simulink model "assignmentJoint"  (R2021b)
settings: Solver=VariableStepAuto  StartTime=0.0  StopTime=10.0  MaxStep=0.02  RelTol=1e-3
settings Model: Creator=emil1  LastModifiedBy=emil1

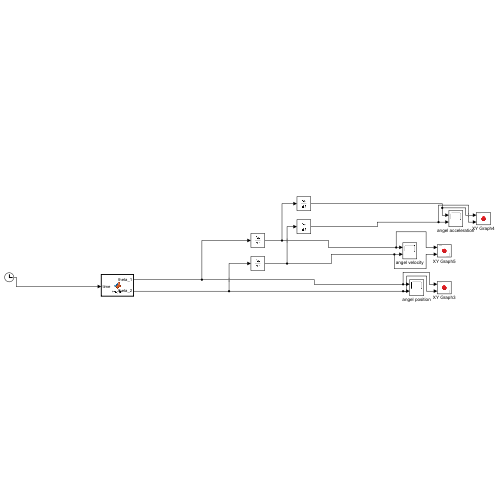
[thumbnail: Simulink's stored preview of the top-level diagram]
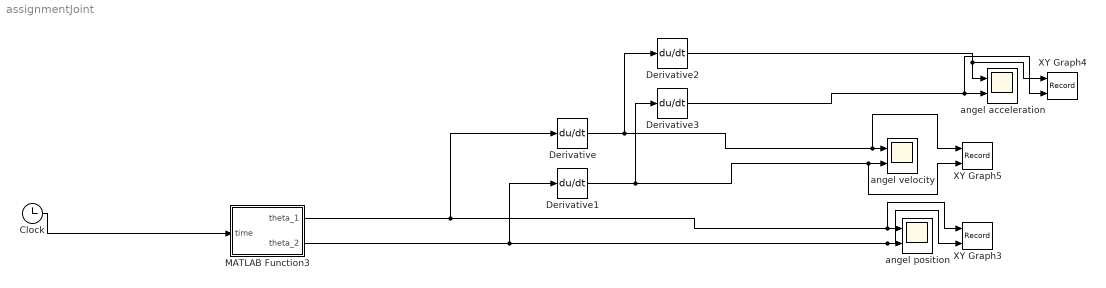
== system assignmentJoint ==
  Clock : Clock
  Derivative{,1..3} (4 alike) : Derivative
  MATLAB Function3 : MATLAB Function  TreatAsAtomicUnit=on
  XY Graph3 : Record  FileSettingsInternal="{\"entries\":[{\"content\":{\"excelSettings\":{\"content\":{},\"type\":\"Streamout.ExcelSettings\"}},\"type\":\"Streamout.FileSettingStorage\",\"uuid\":\"aac29863-c5f3-4fb7-b6fd-b56b9ff78ad2\"}],\"packageUris\":[\"http://schema.mathworks.com/mf0/streamout_blocks/R2020a\"],\"version\":\"1.0\"}"  Layout=[1 1]  SignalsInternal="{\"entries\":[{\"content\":{\"signals\":[{\"content\":{\"blockPath\":[\"untitled2/XY Graph3\"],\"channel\":[],\"dimensions\":[1],\"domain\":\"untitled2/XY Graph3\",\"lineColor\":\"#a2142f\",\"plots\":[1],\"port\":1,\"sid\":[\"\"],\"signalID\":1104,\"signalName\":\"MATLAB Function3:1\"},\"type\":\"RecordBlkView.Signal\",\"uuid\":\"c0351657-4b5f-43d9-835a-4cb54ee66134\"},{\"content\":{\"blockPath\":[\"untitled2/XY Graph3\"],\"channel\":[],\"dimensions\":[1],\"domain\":\"untitled2/XY Graph3\",\"lineColor\":\"#139fff\",\"plots\":[1],\"port\":2,\"sid\":[\"\"],\"signalID\":1108,\"signalName\":\"MATLAB Function3:2\"},\"type\":\"RecordBlkView.Signal\",\"uuid\":\"c0fcede7-449a-4ae5-9ccf-1a3888cdd257\"}]},\"type\":\"RecordBlkView.InputSignals\",\"uuid\":\"e005789e-251b-477d-9ac0-bfcfe427828d\"}],\"packageUris\":[\"http://schema.mathworks.com/mf0/streamout_blocks/R2020a\"],\"version\":\"1.0\"}"  VisualizationBindings="{\"xyplotplugin\":{\"info\":[{\"series\":[{\"bindingParametersList\":[{\"parameter\":\"X-Axis\",\"signalID\":1104,\"signalName\":\"MATLAB Function3:1\"},{\"parameter\":\"Y-Axis\",\"signalID\":1108,\"signalName\":\"MATLAB Function3:2\"}],\"seriesID\":3499}],\"subplotID\":1}]}}"  CompatibilityTag=XY
  XY Graph4 : Record  FileSettingsInternal="{\"entries\":[{\"content\":{\"excelSettings\":{\"content\":{},\"type\":\"Streamout.ExcelSettings\"}},\"type\":\"Streamout.FileSettingStorage\",\"uuid\":\"228e65c6-18a5-40b0-8a31-91b07e16b393\"}],\"packageUris\":[\"http://schema.mathworks.com/mf0/streamout_blocks/R2020a\"],\"version\":\"1.0\"}"  Layout=[1 1]  SignalsInternal="{\"entries\":[{\"content\":{\"signals\":[{\"content\":{\"blockPath\":[\"untitled2/XY Graph4\"],\"channel\":[],\"dimensions\":[1],\"domain\":\"untitled2/XY Graph4\",\"lineColor\":\"#a2142f\",\"plots\":[1],\"port\":1,\"sid\":[\"\"],\"signalID\":1112,\"signalName\":\"Derivative2\"},\"type\":\"RecordBlkView.Signal\",\"uuid\":\"defd5740-cc03-45a0-9e5e-7022539538e1\"},{\"content\":{\"blockPath\":[\"untitled2/XY Graph4\"],\"channel\":[],\"dimensions\":[1],\"domain\":\"untitled2/XY Graph4\",\"lineColor\":\"#139fff\",\"plots\":[1],\"port\":2,\"sid\":[\"\"],\"signalID\":1116,\"signalName\":\"Derivative3\"},\"type\":\"RecordBlkView.Signal\",\"uuid\":\"563bad76-d9df-4018-9cff-6fd36478c7d5\"}]},\"type\":\"RecordBlkView.InputSignals\",\"uuid\":\"ee608da6-8d13-4c6f-a3e1-b72b8fe41bb4\"}],\"packageUris\":[\"http://schema.mathworks.com/mf0/streamout_blocks/R2020a\"],\"version\":\"1.0\"}"  VisualizationBindings="{\"xyplotplugin\":{\"info\":[{\"series\":[{\"bindingParametersList\":[{\"parameter\":\"X-Axis\",\"signalID\":1112,\"signalName\":\"Derivative2\"},{\"parameter\":\"Y-Axis\",\"signalID\":1116,\"signalName\":\"Derivative3\"}],\"seriesID\":62397}],\"subplotID\":1}]}}"  CompatibilityTag=XY
  XY Graph5 : Record  FileSettingsInternal="{\"entries\":[{\"content\":{\"excelSettings\":{\"content\":{},\"type\":\"Streamout.ExcelSettings\"}},\"type\":\"Streamout.FileSettingStorage\",\"uuid\":\"1833a27e-0556-466c-b821-dc9cf6562ba7\"}],\"packageUris\":[\"http://schema.mathworks.com/mf0/streamout_blocks/R2020a\"],\"version\":\"1.0\"}"  Layout=[1 1]  SignalsInternal="{\"entries\":[{\"content\":{\"signals\":[{\"content\":{\"blockPath\":[\"untitled2/XY Graph5\"],\"channel\":[],\"dimensions\":[1],\"domain\":\"untitled2/XY Graph5\",\"lineColor\":\"#a2142f\",\"plots\":[1],\"port\":1,\"sid\":[\"\"],\"signalID\":1120,\"signalName\":\"Derivative\"},\"type\":\"RecordBlkView.Signal\",\"uuid\":\"e36ac0cd-fd08-42fe-a582-6d0da16de171\"},{\"content\":{\"blockPath\":[\"untitled2/XY Graph5\"],\"channel\":[],\"dimensions\":[1],\"domain\":\"untitled2/XY Graph5\",\"lineColor\":\"#139fff\",\"plots\":[1],\"port\":2,\"sid\":[\"\"],\"signalID\":1124,\"signalName\":\"Derivative1\"},\"type\":\"RecordBlkView.Signal\",\"uuid\":\"e36b8e4c-7988-4b3a-9b98-00cf7bdc5192\"}]},\"type\":\"RecordBlkView.InputSignals\",\"uuid\":\"1bbb7466-d6ec-480c-a003-5d6719632f7e\"}],\"packageUris\":[\"http://schema.mathworks.com/mf0/streamout_blocks/R2020a\"],\"version\":\"1.0\"}"  VisualizationBindings="{\"xyplotplugin\":{\"info\":[{\"series\":[{\"bindingParametersList\":[{\"parameter\":\"X-Axis\",\"signalID\":1120,\"signalName\":\"Derivative\"},{\"parameter\":\"Y-Axis\",\"signalID\":1124,\"signalName\":\"Derivative1\"}],\"seriesID\":28726}],\"subplotID\":1}]}}"  CompatibilityTag=XY
  angel acceleration : Scope  NumInputPorts=2
  angel position : Scope  NumInputPorts=2
  angel velocity : Scope  NumInputPorts=2
  wires:
  Clock/1 -> MATLAB Function3/1(time)
  Derivative2/1 -> angel acceleration/1, XY Graph4/1
  Derivative3/1 -> angel acceleration/2, XY Graph4/2
  MATLAB Function3/1(theta_1) -> Derivative/1, XY Graph3/1, angel position/1
  MATLAB Function3/2(theta_2) -> Derivative1/1, XY Graph3/2, angel position/2
  Derivative1/1 -> Derivative3/1, XY Graph5/2, angel velocity/2
  Derivative/1 -> Derivative2/1, XY Graph5/1, angel velocity/1

== matlab function assignmentJoint/MATLAB Function3 ==
  data: theta_1 output; theta_2 output; time input
function [theta_1, theta_2]= theta(time)

radian = pi*45/180;

theta_1 = 3*sin(pi*time);

theta_2 = 0.5*sin(3*pi*time+radian);
